simulink model "AirLevitation_cl_v2"  (R2023a)
settings: Solver=FixedStepDiscrete  StartTime=0.0  StopTime=inf  FixedStep=0.002  RelTol=1e-3  EnableMultiTasking=on
undefined symbols (not defined in the file): DiscIntNeverNeededParam
libraries: arduinolib x3, simulink x1, arduinosensorlib x1, SignalEditorBlockLib x1
settings Model: SimulationMode=external  ExtModeTrigDuration=2  Creator=auw_a  LastModifiedBy=auw_a
settings SolverCC: AlgebraicLoopSolver=TrustRegion  PositivePriorityOrder=on
settings DataIOCC: ReturnWorkspaceOutputs=off
settings OptimizationCC: EnhancedBackFolding=on  PassReuseOutputArgsAs=Individual arguments  ZeroExternalMemoryAtStartup=off  ZeroInternalMemoryAtStartup=off  MaxStackSize=64  OptimizeBlockOrder=speed  DifferentSizesBufferReuse=on  OptimizationCustomize=off  EfficientTunableParamExpr=on
settings DebuggingCC: ParameterTunabilityLossMsg=error  UnconnectedInputMsg=warning  UnconnectedOutputMsg=warning  UnconnectedLineMsg=warning  ArithmeticOperatorsInVariantConditions=warning
settings HardwareCC: ProdBitPerInt=16  ProdBitPerPointer=16  ProdBitPerSizeT=16  ProdBitPerPtrDiffT=16  ProdLargestAtomicFloat=None  ProdWordSize=8  ProdHWDeviceType=Atmel->AVR
settings ModelReferenceCC: EnableRefExpFcnMdlSchedulingChecks=on
settings SFSimCC: SimUseLocalCustomCode=off  MATLABDynamicMemAlloc=off  CustomCodeUndefinedFunction=UseInterfaceOnly
settings RTWCC: Description=Embedded Coder  SystemTargetFile=ert.tlc  HardwareBoard=Arduino Uno  TemplateMakefile=ert_default_tmf  RTWUseLocalCustomCode=off  Toolchain=Arduino AVR  BuildConfiguration=Faster Runs
settings CodeAppCC: ForceParamTrailComments=on  IgnoreCustomStorageClasses=off  OperatorAnnotations=on  SimulinkDataObjDesc=on  SFDataObjDesc=on  InsertBlockDesc=on
settings ERTTargetCC: SupportContinuousTime=on  SupportVariableSizeSignals=on  ExtMode=on  ExtModeTransport=3  ExtModeStaticAlloc=on  ExtModeAutomaticAllocSize=off  ExtModeStaticAllocSize=250  ExtModeMexFile=ext_xcp  ExtModeMexArgs=0 10 115200  ExtModeIntrfLevel=Level2 - Open
settings ConfigComp: CovMetricSettings=dswe

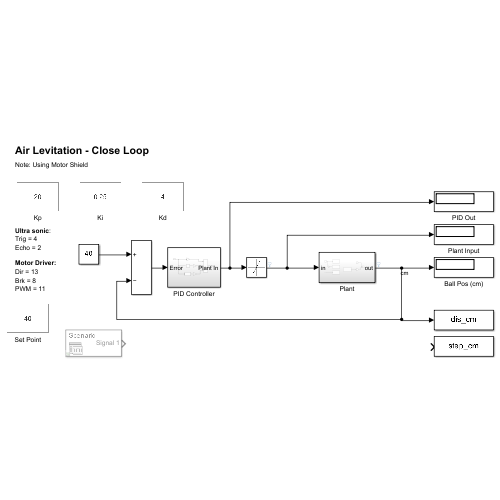
[thumbnail: Simulink's stored preview of the top-level diagram]
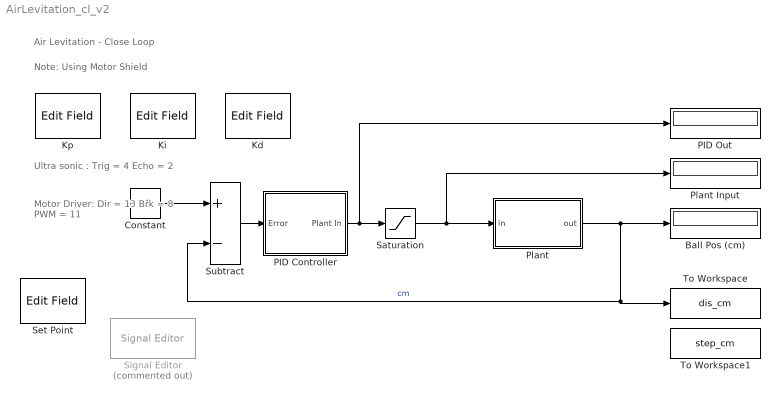
== system AirLevitation_cl_v2 ==
  note: Note: Using Motor Shield
  note: Air Levitation - Close Loop
  note: Motor Driver:
      | Dir = 13
      | Brk = 8
      | PWM = 11
  note: Ultra sonic :
      | Trig = 4
      | Echo = 2
  Ball Pos (cm) : Display
  Constant : Constant  Value=40
  Kd : EditField  LabelPosition=Hide  ShowInitialText=on  Alignment=Center
  Ki : EditField  LabelPosition=Hide  ShowInitialText=on  Alignment=Center
  Kp : EditField  LabelPosition=Hide  ShowInitialText=on  Alignment=Center
  PID Controller : Subsystem
  PID Out : Display
  Plant : Subsystem
  Plant Input : Display
  Saturation : Saturate  UpperLimit=255  LowerLimit=80
  Set Point : EditField  LabelPosition=Hide  ShowInitialText=on  Alignment=Center
  Signal Editor : SignalEditorBlockLib/Signal Editor  Commented=on  FileName=Signal.mat  ActiveScenario=Scenario  ActiveSignal=Signal 1  IsBus=off  OutputBusObjectStr=Bus: BusObject  SampleTime=0.04  Interpolate=off  ZeroCross=off  OutputAfterFinalValue=Setting to zero  Unit=inherit  PreserveSignalName=on  ApplySigPropsToAllScenarios=on
  Subtract : Sum  Inputs=+-
  To Workspace : ToWorkspace  VariableName=dis_cm  SampleTime=-1
      settings: Save2DSignal=2-D array (concatenate along first dimension)
  To Workspace1 : ToWorkspace  VariableName=step_cm  SampleTime=-1
      settings: Save2DSignal=2-D array (concatenate along first dimension)
  wires:
  Plant/1(out) -> To Workspace/1, Subtract/2, Ball Pos (cm)/1  "cm"
  Saturation/1 -> Plant/1(in), Plant Input/1
  PID Controller/1(Plant In) -> Saturation/1, PID Out/1
  Subtract/1 -> PID Controller/1(Error)
  Constant/1 -> Subtract/1

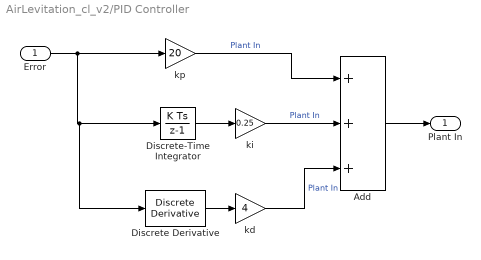
== system AirLevitation_cl_v2/PID Controller ==
  Error : Inport
  Add : Sum  Inputs=+++
  Discrete Derivative : simulink/Discrete/Discrete Derivative  gainval=1.0  ICPrevScaledInput=0.0  OutMin=[]  OutMax=[]  OutDataType=fixdt(1, 16)  OutScaling=2^-10  DoSatur=off
  Discrete-Time Integrator : DiscreteIntegrator  SampleTime=-1  ICPrevOutput=DiscIntNeverNeededParam  ICPrevScaledInput=DiscIntNeverNeededParam
  kd : Gain  Gain=4
  ki : Gain  Gain=0.25
  kp : Gain  Gain=20
  Plant In : Outport
  wires:
  Error/1 -> Discrete Derivative/1, Discrete-Time Integrator/1, kp/1
  Add/1 -> Plant In/1
  kp/1 -> Add/1  "Plant In"
  Discrete-Time Integrator/1 -> ki/1
  Discrete Derivative/1 -> kd/1
  ki/1 -> Add/2  "Plant In"
  kd/1 -> Add/3  "Plant In"

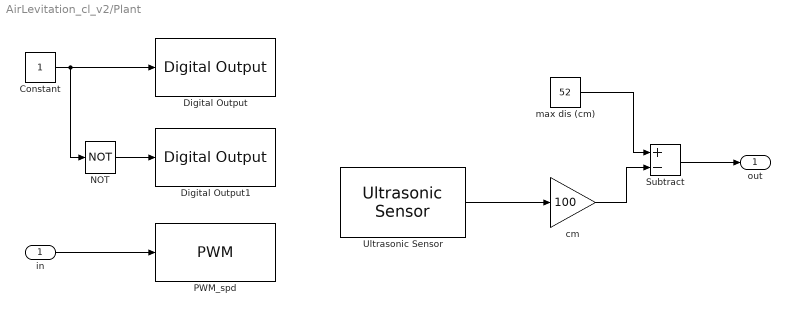
== system AirLevitation_cl_v2/Plant ==
  in : Inport
  Constant : Constant
  Digital Output : arduinolib/Digital Output  pinNumber=13  Direction=output  blockPlatform=arduino
  Digital Output1 : arduinolib/Digital Output  pinNumber=8  Direction=output  blockPlatform=arduino
  NOT : Logic  Operator=NOT  IconShape=distinctive  AllPortsSameDT=off  OutDataTypeStr=boolean
  PWM_spd : arduinolib/PWM  pinNumber=11  frequencyType=Default  desiredFrequency=980.4  achievableFrequency=980.4
  Subtract : Sum  Inputs=+-
  Ultrasonic Sensor : arduinosensorlib/Ultrasonic Sensor  NumSignalPins=2  TrigPin=4  EchoPin=2  SignalPin=3  SampleTime_=0.04  blockPlatform=ARDUINO
  cm : Gain  Gain=100
  max dis (cm) : Constant  Value=52
  out : Outport
  wires:
  in/1 -> PWM_spd/1
  Ultrasonic Sensor/1 -> cm/1
  cm/1 -> Subtract/2
  Subtract/1 -> out/1
  max dis (cm)/1 -> Subtract/1
  NOT/1 -> Digital Output1/1
  Constant/1 -> Digital Output/1, NOT/1
